simulink model "generic_IVS"  (R2024a)
settings: Solver=FixedStepDiscrete  StartTime=0.0  StopTime=inf  FixedStep=0.001  RelTol=1e-3  EnableMultiTasking=on
libraries: CarMaker4SL x52, slpidlib x2, simulink x1
(part 3 of 3)

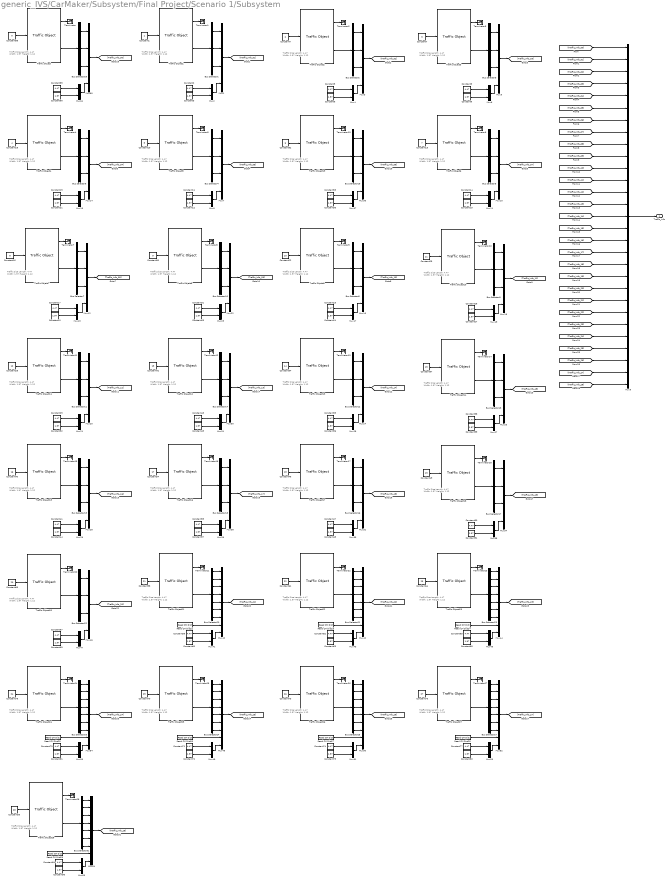
== system generic_IVS/CarMaker/Subsystem/Final Project/Scenario 1/Subsystem ==
  note: Traffic Size
      | Length: 4.47
      | Width: 1.97
      | Height: 1.12
  note: Traffic Size
      | Length: 4.47
      | Width: 1.97
      | Height: 1.12
  note: Traffic Size
      | Length: 4.47
      | Width: 1.97
      | Height: 1.12
  note: Traffic Size
      | Length: 4.47
      | Width: 1.97
      | Height: 1.12
  note: Traffic Size
      | Length: 4.47
      | Width: 1.97
      | Height: 1.12
  note: Traffic Size
      | Length: 4.47
      | Width: 1.97
      | Height: 1.12
  note: Traffic Size
      | Length: 4.47
      | Width: 1.97
      | Height: 1.12
  note: Traffic Size
      | Length: 4.47
      | Width: 1.97
      | Height: 1.12
  note: Traffic Size
      | Length: 4.47
      | Width: 1.97
      | Height: 1.12
  note: Traffic Size
      | Length: 4.47
      | Width: 1.97
      | Height: 1.12
  note: Traffic Size
      | Length: 4.47
      | Width: 1.97
      | Height: 1.12
  note: Traffic Size
      | Length: 4.47
      | Width: 1.97
      | Height: 1.12
  note: Traffic Size
      | Length: 4.47
      | Width: 1.97
      | Height: 1.12
  note: Traffic Size
      | Length: 4.47
      | Width: 1.97
      | Height: 1.12
  note: Traffic Size
      | Length: 4.47
      | Width: 1.97
      | Height: 1.12
  note: Traffic Size
      | Length: 4.47
      | Width: 1.97
      | Height: 1.12
  note: Traffic Size
      | Length: 4.47
      | Width: 1.97
      | Height: 1.12
  note: Traffic Size
      | Length: 4.47
      | Width: 1.97
      | Height: 1.12
  note: Traffic Size
      | Length: 4.47
      | Width: 1.97
      | Height: 1.12
  note: Traffic Size
      | Length: 4.47
      | Width: 1.97
      | Height: 1.12
  note: Traffic Size
      | Length: 4.47
      | Width: 1.97
      | Height: 1.12
  note: Traffic Size
      | Length: 4.47
      | Width: 1.97
      | Height: 1.12
  note: Traffic Size
      | Length: 4.47
      | Width: 1.97
      | Height: 1.12
  note: Traffic Size
      | Length: 4.47
      | Width: 1.97
      | Height: 1.12
  note: Traffic Size
      | Length: 4.47
      | Width: 1.97
      | Height: 1.12
  note: Traffic Size
      | Length: 4.47
      | Width: 1.97
      | Height: 1.12
  note: Traffic Size
      | Length: 4.47
      | Width: 1.97
      | Height: 1.12
  note: Traffic Size
      | Length: 4.47
      | Width: 1.97
      | Height: 1.12
  note: Traffic Size
      | Length: 4.47
      | Width: 1.97
      | Height: 1.12
  Bus Selector{1..19,22,29} (21 alike) : BusSelector  OutputSignals=t_0 x,t_0 y,r_zyx z
  Bus Selector{20..21,23..27,31} (8 alike) : BusSelector  OutputSignals=t_0 x,t_0 y,v_0 x,v_0 y,a_0 x,a_0 y,r_zyx z
  Constant1 : Constant
  Constant10 : Constant  Value=5
  Constant{2,5,8,11,14,17,19,23,26,29,31,35,38,41,43,47,50,53,55,59,62,65,67,71,74,77,79,89,94} (29 alike) : Constant  Value=4.47
  Constant{3,6,9,12,15,20..21,24,27,32..33,36,39,44..45,48,51,56..57,60,63,68..69,72,75,80..81,90,96} (29 alike) : Constant  Value=1.97
  Constant13 : Constant  Value=7
  Constant16 : Constant  Value=8
  Constant18 : Constant  Value=4
  Constant22 : Constant  Value=10
  Constant25 : Constant  Value=11
  Constant28 : Constant  Value=12
  Constant30 : Constant  Value=9
  Constant34 : Constant  Value=14
  Constant37 : Constant  Value=15
  Constant4 : Constant  Value=2
  Constant40 : Constant  Value=16
  Constant42 : Constant  Value=13
  Constant46 : Constant  Value=18
  Constant49 : Constant  Value=19
  Constant52 : Constant  Value=6
  Constant54 : Constant  Value=17
  Constant58 : Constant  Value=21
  Constant61 : Constant  Value=22
  Constant64 : Constant  Value=23
  Constant66 : Constant  Value=20
  Constant7 : Constant  Value=3
  Constant70 : Constant  Value=25
  Constant73 : Constant  Value=26
  Constant76 : Constant  Value=27
  Constant78 : Constant  Value=24
  Constant88 : Constant  Value=0
  Constant93 : Constant  Value=28
  Mux{1,3,5,7,10,12,14,16,18,20,22,24,26,28,30,32,34,36,38,46,60} (21 alike) : Mux
  Mux{2,4,6,8,11,13,15,17,19,21,23,25,27,29,31,33,35,37,39,41,43,45,47,49,51,53,55,61,65} (29 alike) : Mux  Inputs=2
  Mux{40,42,44,48,50,52,54,64} (8 alike) : Mux  Inputs=9
  Mux9 : Mux  Inputs=29
  Read CM Dict22 : CarMaker4SL/Read CM Dict  xname=Traffic.T21.rzv  xsync=off  xstime=Inherited
  Read CM Dict23 : CarMaker4SL/Read CM Dict  xname=Traffic.T22.rzv  xsync=off  xstime=Inherited
  Read CM Dict24 : CarMaker4SL/Read CM Dict  xname=Traffic.T23.rzv  xsync=off  xstime=Inherited
  Read CM Dict25 : CarMaker4SL/Read CM Dict  xname=Traffic.T24.rzv  xsync=off  xstime=Inherited
  Read CM Dict26 : CarMaker4SL/Read CM Dict  xname=Traffic.T25.rzv  xsync=off  xstime=Inherited
  Read CM Dict27 : CarMaker4SL/Read CM Dict  xname=Traffic.T26.rzv  xsync=off  xstime=Inherited
  Read CM Dict28 : CarMaker4SL/Read CM Dict  xname=Traffic.T27.rzv  xsync=off  xstime=Inherited
  Read CM Dict29 : CarMaker4SL/Read CM Dict  xname=Traffic.T28.rzv  xsync=off  xstime=Inherited
  Terminator{,1..28} (29 alike) : Terminator
  Traffic Object : CarMaker4SL/Traffic Object  xname=T00  ximode=Traffic Id  xstime=Inherited
      settings: SourceProductName=CarMaker4SL
  Traffic Object1 : CarMaker4SL/Traffic Object  xname=T01  ximode=Traffic Id  xstime=Inherited
      settings: SourceProductName=CarMaker4SL
  Traffic Object10 : CarMaker4SL/Traffic Object  xname=T11  ximode=Traffic Id  xstime=Inherited
      settings: SourceProductName=CarMaker4SL
  Traffic Object11 : CarMaker4SL/Traffic Object  xname=T12  ximode=Traffic Id  xstime=Inherited
      settings: SourceProductName=CarMaker4SL
  Traffic Object12 : CarMaker4SL/Traffic Object  xname=T13  ximode=Traffic Id  xstime=Inherited
      settings: SourceProductName=CarMaker4SL
  Traffic Object13 : CarMaker4SL/Traffic Object  xname=T14  ximode=Traffic Id  xstime=Inherited
      settings: SourceProductName=CarMaker4SL
  Traffic Object14 : CarMaker4SL/Traffic Object  xname=T15  ximode=Traffic Id  xstime=Inherited
      settings: SourceProductName=CarMaker4SL
  Traffic Object15 : CarMaker4SL/Traffic Object  xname=T16  ximode=Traffic Id  xstime=Inherited
      settings: SourceProductName=CarMaker4SL
  Traffic Object16 : CarMaker4SL/Traffic Object  xname=T17  ximode=Traffic Id  xstime=Inherited
      settings: SourceProductName=CarMaker4SL
  Traffic Object17 : CarMaker4SL/Traffic Object  xname=T18  ximode=Traffic Id  xstime=Inherited
      settings: SourceProductName=CarMaker4SL
  Traffic Object18 : CarMaker4SL/Traffic Object  xname=T19  ximode=Traffic Id  xstime=Inherited
      settings: SourceProductName=CarMaker4SL
  Traffic Object19 : CarMaker4SL/Traffic Object  xname=T06  ximode=Traffic Id  xstime=Inherited
      settings: SourceProductName=CarMaker4SL
  Traffic Object2 : CarMaker4SL/Traffic Object  xname=T02  ximode=Traffic Id  xstime=Inherited
      settings: SourceProductName=CarMaker4SL
  Traffic Object20 : CarMaker4SL/Traffic Object  xname=T20  ximode=Traffic Id  xstime=Inherited
      settings: SourceProductName=CarMaker4SL
  Traffic Object21 : CarMaker4SL/Traffic Object  xname=T21  ximode=Traffic Id  xstime=Inherited
      settings: SourceProductName=CarMaker4SL
  Traffic Object22 : CarMaker4SL/Traffic Object  xname=T22  ximode=Traffic Id  xstime=Inherited
      settings: SourceProductName=CarMaker4SL
  Traffic Object23 : CarMaker4SL/Traffic Object  xname=T23  ximode=Traffic Id  xstime=Inherited
      settings: SourceProductName=CarMaker4SL
  Traffic Object24 : CarMaker4SL/Traffic Object  xname=T24  ximode=Traffic Id  xstime=Inherited
      settings: SourceProductName=CarMaker4SL
  Traffic Object25 : CarMaker4SL/Traffic Object  xname=T25  ximode=Traffic Id  xstime=Inherited
      settings: SourceProductName=CarMaker4SL
  Traffic Object26 : CarMaker4SL/Traffic Object  xname=T26  ximode=Traffic Id  xstime=Inherited
      settings: SourceProductName=CarMaker4SL
  Traffic Object27 : CarMaker4SL/Traffic Object  xname=T27  ximode=Traffic Id  xstime=Inherited
      settings: SourceProductName=CarMaker4SL
  Traffic Object28 : CarMaker4SL/Traffic Object  xname=T28  ximode=Traffic Id  xstime=Inherited
      settings: SourceProductName=CarMaker4SL
  Traffic Object3 : CarMaker4SL/Traffic Object  xname=T03  ximode=Traffic Id  xstime=Inherited
      settings: SourceProductName=CarMaker4SL
  Traffic Object4 : CarMaker4SL/Traffic Object  xname=T04  ximode=Traffic Id  xstime=Inherited
      settings: SourceProductName=CarMaker4SL
  Traffic Object5 : CarMaker4SL/Traffic Object  xname=T05  ximode=Traffic Id  xstime=Inherited
      settings: SourceProductName=CarMaker4SL
  Traffic Object6 : CarMaker4SL/Traffic Object  xname=T07  ximode=Traffic Id  xstime=Inherited
      settings: SourceProductName=CarMaker4SL
  Traffic Object7 : CarMaker4SL/Traffic Object  xname=T08  ximode=Traffic Id  xstime=Inherited
      settings: SourceProductName=CarMaker4SL
  Traffic Object8 : CarMaker4SL/Traffic Object  xname=T09  ximode=Traffic Id  xstime=Inherited
      settings: SourceProductName=CarMaker4SL
  Traffic Object9 : CarMaker4SL/Traffic Object  xname=T10  ximode=Traffic Id  xstime=Inherited
      settings: SourceProductName=CarMaker4SL
  Traffic_Info : Outport
  wires:
  [Traffic_Info_00] -> Mux9/1
  [Traffic_Info_01] -> Mux9/2
  Mux9/1 -> Traffic_Info/1
  [Traffic_Info_02] -> Mux9/3
  [Traffic_Info_06] -> Mux9/7
  [Traffic_Info_05] -> Mux9/6
  [Traffic_Info_04] -> Mux9/5
  [Traffic_Info_03] -> Mux9/4
  [Traffic_Info_09] -> Mux9/10
  [Traffic_Info_10] -> Mux9/11
  [Traffic_Info_11] -> Mux9/12
  [Traffic_Info_08] -> Mux9/9
  [Traffic_Info_12] -> Mux9/13
  [Traffic_Info_13] -> Mux9/14
  [Traffic_Info_07] -> Mux9/8
  [Traffic_Info_16] -> Mux9/17
  [Traffic_Info_17] -> Mux9/18
  [Traffic_Info_18] -> Mux9/19
  [Traffic_Info_15] -> Mux9/16
  [Traffic_Info_19] -> Mux9/20
  [Traffic_Info_20] -> Mux9/21
  [Traffic_Info_14] -> Mux9/15
  [Traffic_Info_23] -> Mux9/24
  [Traffic_Info_24] -> Mux9/25
  [Traffic_Info_25] -> Mux9/26
  [Traffic_Info_22] -> Mux9/23
  [Traffic_Info_26] -> Mux9/27
  [Traffic_Info_27] -> Mux9/28
  [Traffic_Info_21] -> Mux9/22
  [Traffic_Info_28] -> Mux9/29
  Traffic Object/2 -> Bus Selector29/1
  Constant88/1 -> Traffic Object/1
  Traffic Object/1 -> Terminator/1
  Bus Selector29/1 -> Mux60/1  "<t_0 x>"
  Bus Selector29/2 -> Mux60/2  "<t_0 y>"
  Bus Selector29/3 -> Mux60/3  "<r_zyx z>"
  Mux60/1 -> [Traffic_Info_00]
  Constant89/1 -> Mux61/1
  Constant90/1 -> Mux61/2
  Mux61/1 -> Mux60/4
  Bus Selector23/5 -> Mux44/5  "<a_0 x>"
  Traffic Object22/2 -> Bus Selector21/1
  Mux41/1 -> Mux40/9
  Constant63/1 -> Mux43/2
  Bus Selector23/2 -> Mux44/2  "<t_0 y>"
  Bus Selector21/2 -> Mux42/2  "<t_0 y>"
  Bus Selector21/5 -> Mux42/5  "<a_0 x>"
  Traffic Object22/1 -> Terminator22/1
  Bus Selector23/6 -> Mux44/6  "<a_0 y>"
  Bus Selector23/7 -> Mux44/7  "<r_zyx z>"
  Traffic Object23/1 -> Terminator23/1
  Traffic Object23/2 -> Bus Selector23/1
  Constant68/1 -> Mux45/2
  Mux45/1 -> Mux44/9
  Constant61/1 -> Traffic Object22/1
  Read CM Dict24/1 -> Mux44/8
  Mux42/1 -> [Traffic_Info_22]
  Mux40/1 -> [Traffic_Info_21]
  Mux44/1 -> [Traffic_Info_23]
  Bus Selector23/4 -> Mux44/4  "<v_0 y>"
  Bus Selector21/6 -> Mux42/6  "<a_0 y>"
  Bus Selector20/6 -> Mux40/6  "<a_0 y>"
  Bus Selector21/3 -> Mux42/3  "<v_0 x>"
  Bus Selector21/4 -> Mux42/4  "<v_0 y>"
  Bus Selector21/1 -> Mux42/1  "<t_0 x>"
  Constant58/1 -> Traffic Object21/1
  Bus Selector21/7 -> Mux42/7  "<r_zyx z>"
  Constant65/1 -> Mux45/1
  Bus Selector20/1 -> Mux40/1  "<t_0 x>"
  Bus Selector23/1 -> Mux44/1  "<t_0 x>"
  Bus Selector20/3 -> Mux40/3  "<v_0 x>"
  Constant60/1 -> Mux41/2
  Traffic Object21/2 -> Bus Selector20/1
  Read CM Dict22/1 -> Mux40/8
  Bus Selector20/5 -> Mux40/5  "<a_0 x>"
  Traffic Object21/1 -> Terminator21/1
  Bus Selector20/2 -> Mux40/2  "<t_0 y>"
  Bus Selector23/3 -> Mux44/3  "<v_0 x>"
  Constant64/1 -> Traffic Object23/1
  Bus Selector20/7 -> Mux40/7  "<r_zyx z>"
  Read CM Dict23/1 -> Mux42/8
  Constant62/1 -> Mux43/1
  Bus Selector20/4 -> Mux40/4  "<v_0 y>"
  Constant59/1 -> Mux41/1
  Mux43/1 -> Mux42/9
  Bus Selector26/3 -> Mux54/3  "<v_0 x>"
  Bus Selector27/5 -> Mux52/5  "<a_0 x>"
  Bus Selector26/5 -> Mux54/5  "<a_0 x>"
  Traffic Object26/2 -> Bus Selector25/1
  Bus Selector26/6 -> Mux54/6  "<a_0 y>"
  Mux49/1 -> Mux48/9
  Constant75/1 -> Mux51/2
  Bus Selector27/2 -> Mux52/2  "<t_0 y>"
  Bus Selector25/2 -> Mux50/2  "<t_0 y>"
  Bus Selector25/5 -> Mux50/5  "<a_0 x>"
  Traffic Object26/1 -> Terminator26/1
  Bus Selector27/6 -> Mux52/6  "<a_0 y>"
  Bus Selector26/7 -> Mux54/7  "<r_zyx z>"
  Bus Selector27/7 -> Mux52/7  "<r_zyx z>"
  Bus Selector26/1 -> Mux54/1  "<t_0 x>"
  Traffic Object27/1 -> Terminator27/1
  Traffic Object27/2 -> Bus Selector27/1
  Constant80/1 -> Mux53/2
  Mux53/1 -> Mux52/9
  Constant73/1 -> Traffic Object26/1
  Read CM Dict28/1 -> Mux52/8
  Mux50/1 -> [Traffic_Info_26]
  Mux48/1 -> [Traffic_Info_25]
  Mux52/1 -> [Traffic_Info_27]
  Bus Selector27/4 -> Mux52/4  "<v_0 y>"
  Constant78/1 -> Traffic Object24/1
  Traffic Object24/1 -> Terminator24/1
  Bus Selector25/6 -> Mux50/6  "<a_0 y>"
  Bus Selector24/6 -> Mux48/6  "<a_0 y>"
  Bus Selector25/3 -> Mux50/3  "<v_0 x>"
  Read CM Dict25/1 -> Mux54/8
  Bus Selector25/4 -> Mux50/4  "<v_0 y>"
  Bus Selector26/4 -> Mux54/4  "<v_0 y>"
  Bus Selector25/1 -> Mux50/1  "<t_0 x>"
  Constant70/1 -> Traffic Object25/1
  Bus Selector25/7 -> Mux50/7  "<r_zyx z>"
  Constant77/1 -> Mux53/1
  Bus Selector26/2 -> Mux54/2  "<t_0 y>"
  Bus Selector24/1 -> Mux48/1  "<t_0 x>"
  Bus Selector27/1 -> Mux52/1  "<t_0 x>"
  Bus Selector24/3 -> Mux48/3  "<v_0 x>"
  Mux54/1 -> [Traffic_Info_24]
  Constant72/1 -> Mux49/2
  Traffic Object25/2 -> Bus Selector24/1
  Read CM Dict26/1 -> Mux48/8
  Bus Selector24/5 -> Mux48/5  "<a_0 x>"
  Traffic Object25/1 -> Terminator25/1
  Constant81/1 -> Mux55/2
  Bus Selector24/2 -> Mux48/2  "<t_0 y>"
  Bus Selector27/3 -> Mux52/3  "<v_0 x>"
  Constant76/1 -> Traffic Object27/1
  Bus Selector24/7 -> Mux48/7  "<r_zyx z>"
  Traffic Object24/2 -> Bus Selector26/1
  Read CM Dict27/1 -> Mux50/8
  Mux55/1 -> Mux54/9
  Constant74/1 -> Mux51/1
  Bus Selector24/4 -> Mux48/4  "<v_0 y>"
  Constant71/1 -> Mux49/1
  Constant79/1 -> Mux55/1
  Mux51/1 -> Mux50/9
  Bus Selector31/3 -> Mux64/3  "<v_0 x>"
  Bus Selector31/5 -> Mux64/5  "<a_0 x>"
  Bus Selector31/6 -> Mux64/6  "<a_0 y>"
  Bus Selector31/7 -> Mux64/7  "<r_zyx z>"
  Bus Selector31/1 -> Mux64/1  "<t_0 x>"
  Constant93/1 -> Traffic Object28/1
  Traffic Object28/1 -> Terminator28/1
  Read CM Dict29/1 -> Mux64/8
  Bus Selector31/4 -> Mux64/4  "<v_0 y>"
  Bus Selector31/2 -> Mux64/2  "<t_0 y>"
  Mux64/1 -> [Traffic_Info_28]
  Constant96/1 -> Mux65/2
  Traffic Object28/2 -> Bus Selector31/1
  Mux65/1 -> Mux64/9
  Constant94/1 -> Mux65/1
  Bus Selector1/3 -> Mux1/3  "<r_zyx z>"
  Mux1/1 -> [Traffic_Info_01]
  Bus Selector1/1 -> Mux1/1  "<t_0 x>"
  Traffic Object1/1 -> Terminator1/1
  Constant2/1 -> Mux2/1
  Constant3/1 -> Mux2/2
  Bus Selector1/2 -> Mux1/2  "<t_0 y>"
  Mux2/1 -> Mux1/4
  Constant1/1 -> Traffic Object1/1
  Traffic Object1/2 -> Bus Selector1/1
  Bus Selector2/3 -> Mux3/3  "<r_zyx z>"
  Mux3/1 -> [Traffic_Info_02]
  Bus Selector2/1 -> Mux3/1  "<t_0 x>"
  Traffic Object2/1 -> Terminator2/1
  Constant5/1 -> Mux4/1
  Constant6/1 -> Mux4/2
  Bus Selector2/2 -> Mux3/2  "<t_0 y>"
  Mux4/1 -> Mux3/4
  Constant4/1 -> Traffic Object2/1
  Traffic Object2/2 -> Bus Selector2/1
  Bus Selector3/3 -> Mux5/3  "<r_zyx z>"
  Mux5/1 -> [Traffic_Info_03]
  Bus Selector3/1 -> Mux5/1  "<t_0 x>"
  Traffic Object3/1 -> Terminator3/1
  Constant8/1 -> Mux6/1
  Constant9/1 -> Mux6/2
  Bus Selector3/2 -> Mux5/2  "<t_0 y>"
  Mux6/1 -> Mux5/4
  Constant7/1 -> Traffic Object3/1
  Traffic Object3/2 -> Bus Selector3/1
  Bus Selector6/3 -> Mux14/3  "<r_zyx z>"
  Mux14/1 -> [Traffic_Info_04]
  Bus Selector6/1 -> Mux14/1  "<t_0 x>"
  Mux8/1 -> Mux7/4
  Constant12/1 -> Mux8/2
  Mux7/1 -> [Traffic_Info_05]
  Traffic Object4/1 -> Terminator4/1
  Bus Selector4/2 -> Mux7/2  "<t_0 y>"
  Constant18/1 -> Traffic Object4/1
  Constant21/1 -> Mux15/2
  Constant10/1 -> Traffic Object5/1
  Bus Selector6/2 -> Mux14/2  "<t_0 y>"
  Mux15/1 -> Mux14/4
  Traffic Object4/2 -> Bus Selector6/1
  Constant16/1 -> Traffic Object7/1
  Traffic Object7/2 -> Bus Selector7/1
  Constant17/1 -> Mux13/1
  Constant19/1 -> Mux15/1
  Constant11/1 -> Mux8/1
  Traffic Object7/1 -> Terminator7/1
  Constant20/1 -> Mux13/2
  Bus Selector4/1 -> Mux7/1  "<t_0 x>"
  Mux13/1 -> Mux12/4
  Bus Selector7/1 -> Mux12/1  "<t_0 x>"
  Bus Selector4/3 -> Mux7/3  "<r_zyx z>"
  Bus Selector7/3 -> Mux12/3  "<r_zyx z>"
  Mux12/1 -> [Traffic_Info_08]
  Constant15/1 -> Mux11/2
  Mux11/1 -> Mux10/4
  Constant13/1 -> Traffic Object6/1
  Traffic Object5/1 -> Terminator5/1
  Constant14/1 -> Mux11/1
  Traffic Object6/1 -> Terminator6/1
  Traffic Object5/2 -> Bus Selector4/1
  Bus Selector5/1 -> Mux10/1  "<t_0 x>"
  Bus Selector7/2 -> Mux12/2  "<t_0 y>"
  Traffic Object6/2 -> Bus Selector5/1
  Bus Selector5/3 -> Mux10/3  "<r_zyx z>"
  Mux10/1 -> [Traffic_Info_07]
  Bus Selector5/2 -> Mux10/2  "<t_0 y>"
  Bus Selector10/3 -> Mux22/3  "<r_zyx z>"
  Mux22/1 -> [Traffic_Info_09]
  Bus Selector10/1 -> Mux22/1  "<t_0 x>"
  Mux17/1 -> Mux16/4
  Constant24/1 -> Mux17/2
  Mux16/1 -> [Traffic_Info_10]
  Traffic Object8/1 -> Terminator8/1
  Bus Selector8/2 -> Mux16/2  "<t_0 y>"
  Constant30/1 -> Traffic Object8/1
  Constant33/1 -> Mux23/2
  Constant22/1 -> Traffic Object9/1
  Bus Selector10/2 -> Mux22/2  "<t_0 y>"
  Mux23/1 -> Mux22/4
  Traffic Object8/2 -> Bus Selector10/1
  Constant28/1 -> Traffic Object11/1
  Traffic Object11/2 -> Bus Selector11/1
  Constant29/1 -> Mux21/1
  Constant31/1 -> Mux23/1
  Constant23/1 -> Mux17/1
  Traffic Object11/1 -> Terminator11/1
  Constant32/1 -> Mux21/2
  Bus Selector8/1 -> Mux16/1  "<t_0 x>"
  Mux21/1 -> Mux20/4
  Bus Selector11/1 -> Mux20/1  "<t_0 x>"
  Bus Selector8/3 -> Mux16/3  "<r_zyx z>"
  Bus Selector11/3 -> Mux20/3  "<r_zyx z>"
  Mux20/1 -> [Traffic_Info_12]
  Constant27/1 -> Mux19/2
  Mux19/1 -> Mux18/4
  Constant25/1 -> Traffic Object10/1
  Traffic Object9/1 -> Terminator9/1
  Constant26/1 -> Mux19/1
  Traffic Object10/1 -> Terminator10/1
  Traffic Object9/2 -> Bus Selector8/1
  Bus Selector9/1 -> Mux18/1  "<t_0 x>"
  Bus Selector11/2 -> Mux20/2  "<t_0 y>"
  Traffic Object10/2 -> Bus Selector9/1
  Bus Selector9/3 -> Mux18/3  "<r_zyx z>"
  Mux18/1 -> [Traffic_Info_11]
  Bus Selector9/2 -> Mux18/2  "<t_0 y>"
  Bus Selector14/3 -> Mux30/3  "<r_zyx z>"
  Mux30/1 -> [Traffic_Info_13]
  Bus Selector14/1 -> Mux30/1  "<t_0 x>"
  Mux25/1 -> Mux24/4
  Constant36/1 -> Mux25/2
  Mux24/1 -> [Traffic_Info_14]
  Traffic Object12/1 -> Terminator12/1
  Bus Selector12/2 -> Mux24/2  "<t_0 y>"
  Constant42/1 -> Traffic Object12/1
  Constant45/1 -> Mux31/2
  Constant34/1 -> Traffic Object13/1
  Bus Selector14/2 -> Mux30/2  "<t_0 y>"
  Mux31/1 -> Mux30/4
  Traffic Object12/2 -> Bus Selector14/1
  Constant40/1 -> Traffic Object15/1
  Traffic Object15/2 -> Bus Selector15/1
  Constant41/1 -> Mux29/1
  Constant43/1 -> Mux31/1
  Constant35/1 -> Mux25/1
  Traffic Object15/1 -> Terminator15/1
  Constant44/1 -> Mux29/2
  Bus Selector12/1 -> Mux24/1  "<t_0 x>"
  Mux29/1 -> Mux28/4
  Bus Selector15/1 -> Mux28/1  "<t_0 x>"
  Bus Selector12/3 -> Mux24/3  "<r_zyx z>"
  Bus Selector15/3 -> Mux28/3  "<r_zyx z>"
  Mux28/1 -> [Traffic_Info_16]
  Constant39/1 -> Mux27/2
  Mux27/1 -> Mux26/4
  Constant37/1 -> Traffic Object14/1
  Traffic Object13/1 -> Terminator13/1
  Constant38/1 -> Mux27/1
  Traffic Object14/1 -> Terminator14/1
  Traffic Object13/2 -> Bus Selector12/1
  Bus Selector13/1 -> Mux26/1  "<t_0 x>"
  Bus Selector15/2 -> Mux28/2  "<t_0 y>"
  Traffic Object14/2 -> Bus Selector13/1
  Bus Selector13/3 -> Mux26/3  "<r_zyx z>"
  Mux26/1 -> [Traffic_Info_15]
  Bus Selector13/2 -> Mux26/2  "<t_0 y>"
  Bus Selector17/1 -> Mux34/1  "<t_0 x>"
  Traffic Object18/1 -> Terminator18/1
  Constant49/1 -> Traffic Object18/1
  Traffic Object17/2 -> Bus Selector16/1
  Traffic Object17/1 -> Terminator17/1
  Mux34/1 -> [Traffic_Info_19]
  Bus Selector17/3 -> Mux34/3  "<r_zyx z>"
  Constant50/1 -> Mux35/1
  Constant51/1 -> Mux35/2
  Traffic Object18/2 -> Bus Selector17/1
  Constant55/1 -> Mux39/1
  Bus Selector17/2 -> Mux34/2  "<t_0 y>"
  Constant47/1 -> Mux33/1
  Bus Selector16/1 -> Mux32/1  "<t_0 x>"
  Bus Selector16/3 -> Mux32/3  "<r_zyx z>"
  Traffic Object16/2 -> Bus Selector18/1
  Mux39/1 -> Mux38/4
  Constant46/1 -> Traffic Object17/1
  Mux35/1 -> Mux34/4
  Mux32/1 -> [Traffic_Info_18]
  Constant54/1 -> Traffic Object16/1
  Traffic Object16/1 -> Terminator16/1
  Constant48/1 -> Mux33/2
  Mux33/1 -> Mux32/4
  Constant57/1 -> Mux39/2
  Bus Selector18/1 -> Mux38/1  "<t_0 x>"
  Bus Selector18/3 -> Mux38/3  "<r_zyx z>"
  Bus Selector16/2 -> Mux32/2  "<t_0 y>"
  Mux38/1 -> [Traffic_Info_17]
  Bus Selector18/2 -> Mux38/2  "<t_0 y>"
  Bus Selector19/1 -> Mux36/1  "<t_0 x>"
  Traffic Object19/1 -> Terminator19/1
  Constant53/1 -> Mux37/1
  Bus Selector19/2 -> Mux36/2  "<t_0 y>"
  Mux36/1 -> [Traffic_Info_06]
  Bus Selector19/3 -> Mux36/3  "<r_zyx z>"
  Traffic Object19/2 -> Bus Selector19/1
  Mux37/1 -> Mux36/4
  Constant52/1 -> Traffic Object19/1
  Constant56/1 -> Mux37/2
  Constant69/1 -> Mux47/2
  Traffic Object20/2 -> Bus Selector22/1
  Bus Selector22/2 -> Mux46/2  "<t_0 y>"
  Bus Selector22/3 -> Mux46/3  "<r_zyx z>"
  Mux46/1 -> [Traffic_Info_20]
  Constant67/1 -> Mux47/1
  Mux47/1 -> Mux46/4
  Bus Selector22/1 -> Mux46/1  "<t_0 x>"
  Constant66/1 -> Traffic Object20/1
  Traffic Object20/1 -> Terminator20/1

== system generic_IVS/CarMaker/IPG Vehicle/CarAndTrailer/Forces/Suspension Forces/Suspension External Forces Update ==
  Bus Creator21 : BusCreator  Inputs=6
  Bus Creator22 : BusCreator  Inputs=4
  Bus Creator23 : BusCreator  Inputs=4
  From : From  TagVisibility=global
  Ground{32..39} (8 alike) : Ground
  Out1 : Outport
  wires:
  [D] -> Bus Creator21/4
  Ground36/1 -> Bus Creator22/1
  From/1 -> Bus Creator21/1
  [B] -> Bus Creator21/2
  Ground34/1 -> Bus Creator23/3
  Ground32/1 -> Bus Creator23/1
  [C] -> Bus Creator21/3
  Bus Creator23/1 -> Bus Creator21/5
  Ground33/1 -> Bus Creator23/2
  Bus Creator22/1 -> Bus Creator21/6
  Bus Creator21/1 -> Out1/1
  Ground35/1 -> Bus Creator23/4
  Ground39/1 -> Bus Creator22/4
  Ground38/1 -> Bus Creator22/3
  Ground37/1 -> Bus Creator22/2

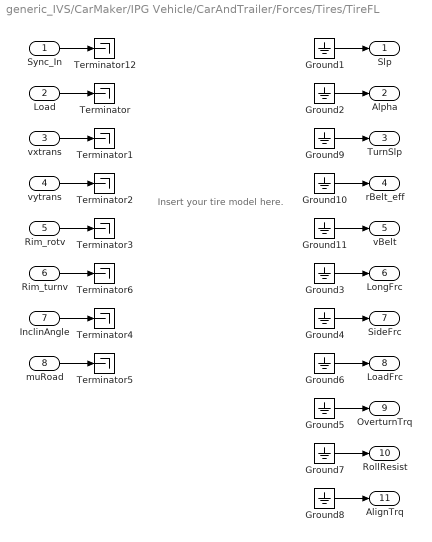
== system generic_IVS/CarMaker/IPG Vehicle/CarAndTrailer/Forces/Tires/TireFL ==
  note: Insert your tire model here.
  Sync_In : Inport
  Load : Inport  Port=2
  vxtrans : Inport  Port=3
  vytrans : Inport  Port=4
  Rim_rotv : Inport  Port=5
  Rim_turnv : Inport  Port=6
  InclinAngle : Inport  Port=7
  muRoad : Inport  Port=8
  Ground{1..11} (11 alike) : Ground
  Terminator{,1..6,12} (8 alike) : Terminator
  Slp : Outport  VectorParamsAs1DForOutWhenUnconnected=off
  Alpha : Outport  Port=2  VectorParamsAs1DForOutWhenUnconnected=off
  TurnSlp : Outport  Port=3  VectorParamsAs1DForOutWhenUnconnected=off
  rBelt_eff : Outport  Port=4  VectorParamsAs1DForOutWhenUnconnected=off
  vBelt : Outport  Port=5  VectorParamsAs1DForOutWhenUnconnected=off
  LongFrc : Outport  Port=6  VectorParamsAs1DForOutWhenUnconnected=off
  SideFrc : Outport  Port=7  VectorParamsAs1DForOutWhenUnconnected=off
  LoadFrc : Outport  Port=8  VectorParamsAs1DForOutWhenUnconnected=off
  OverturnTrq : Outport  Port=9  VectorParamsAs1DForOutWhenUnconnected=off
  RollResist : Outport  Port=10  VectorParamsAs1DForOutWhenUnconnected=off
  AlignTrq : Outport  Port=11  VectorParamsAs1DForOutWhenUnconnected=off
  wires:
  Ground11/1 -> vBelt/1
  Ground10/1 -> rBelt_eff/1
  Ground9/1 -> TurnSlp/1
  Rim_turnv/1 -> Terminator6/1
  Sync_In/1 -> Terminator12/1
  Ground2/1 -> Alpha/1
  Ground3/1 -> LongFrc/1
  Ground4/1 -> SideFrc/1
  Ground5/1 -> OverturnTrq/1
  vxtrans/1 -> Terminator1/1
  vytrans/1 -> Terminator2/1
  Rim_rotv/1 -> Terminator3/1
  InclinAngle/1 -> Terminator4/1
  muRoad/1 -> Terminator5/1
  Load/1 -> Terminator/1
  Ground1/1 -> Slp/1
  Ground6/1 -> LoadFrc/1
  Ground7/1 -> RollResist/1
  Ground8/1 -> AlignTrq/1

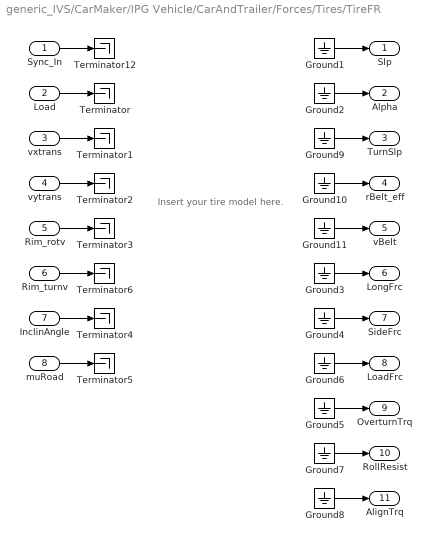
== system generic_IVS/CarMaker/IPG Vehicle/CarAndTrailer/Forces/Tires/TireFR ==
  note: Insert your tire model here.
  Sync_In : Inport
  Load : Inport  Port=2
  vxtrans : Inport  Port=3
  vytrans : Inport  Port=4
  Rim_rotv : Inport  Port=5
  Rim_turnv : Inport  Port=6
  InclinAngle : Inport  Port=7
  muRoad : Inport  Port=8
  Ground{1..11} (11 alike) : Ground
  Terminator{,1..6,12} (8 alike) : Terminator
  Slp : Outport  VectorParamsAs1DForOutWhenUnconnected=off
  Alpha : Outport  Port=2  VectorParamsAs1DForOutWhenUnconnected=off
  TurnSlp : Outport  Port=3  VectorParamsAs1DForOutWhenUnconnected=off
  rBelt_eff : Outport  Port=4  VectorParamsAs1DForOutWhenUnconnected=off
  vBelt : Outport  Port=5  VectorParamsAs1DForOutWhenUnconnected=off
  LongFrc : Outport  Port=6  VectorParamsAs1DForOutWhenUnconnected=off
  SideFrc : Outport  Port=7  VectorParamsAs1DForOutWhenUnconnected=off
  LoadFrc : Outport  Port=8  VectorParamsAs1DForOutWhenUnconnected=off
  OverturnTrq : Outport  Port=9  VectorParamsAs1DForOutWhenUnconnected=off
  RollResist : Outport  Port=10  VectorParamsAs1DForOutWhenUnconnected=off
  AlignTrq : Outport  Port=11  VectorParamsAs1DForOutWhenUnconnected=off
  wires:
  Ground11/1 -> vBelt/1
  Ground10/1 -> rBelt_eff/1
  Ground9/1 -> TurnSlp/1
  Rim_turnv/1 -> Terminator6/1
  Sync_In/1 -> Terminator12/1
  Ground2/1 -> Alpha/1
  Ground3/1 -> LongFrc/1
  Ground4/1 -> SideFrc/1
  Ground5/1 -> OverturnTrq/1
  vxtrans/1 -> Terminator1/1
  vytrans/1 -> Terminator2/1
  Rim_rotv/1 -> Terminator3/1
  InclinAngle/1 -> Terminator4/1
  muRoad/1 -> Terminator5/1
  Load/1 -> Terminator/1
  Ground1/1 -> Slp/1
  Ground6/1 -> LoadFrc/1
  Ground7/1 -> RollResist/1
  Ground8/1 -> AlignTrq/1

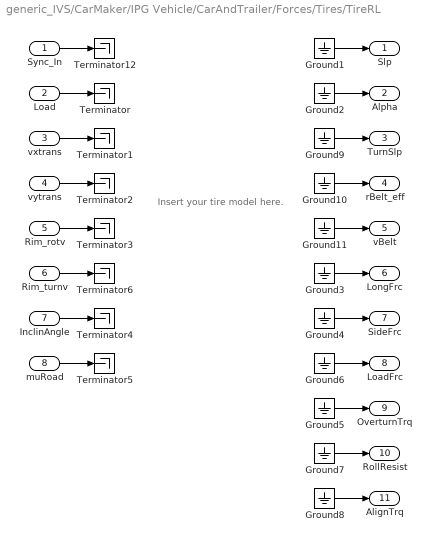
== system generic_IVS/CarMaker/IPG Vehicle/CarAndTrailer/Forces/Tires/TireRL ==
  note: Insert your tire model here.
  Sync_In : Inport
  Load : Inport  Port=2
  vxtrans : Inport  Port=3
  vytrans : Inport  Port=4
  Rim_rotv : Inport  Port=5
  Rim_turnv : Inport  Port=6
  InclinAngle : Inport  Port=7
  muRoad : Inport  Port=8
  Ground{1..11} (11 alike) : Ground
  Terminator{,1..6,12} (8 alike) : Terminator
  Slp : Outport  VectorParamsAs1DForOutWhenUnconnected=off
  Alpha : Outport  Port=2  VectorParamsAs1DForOutWhenUnconnected=off
  TurnSlp : Outport  Port=3  VectorParamsAs1DForOutWhenUnconnected=off
  rBelt_eff : Outport  Port=4  VectorParamsAs1DForOutWhenUnconnected=off
  vBelt : Outport  Port=5  VectorParamsAs1DForOutWhenUnconnected=off
  LongFrc : Outport  Port=6  VectorParamsAs1DForOutWhenUnconnected=off
  SideFrc : Outport  Port=7  VectorParamsAs1DForOutWhenUnconnected=off
  LoadFrc : Outport  Port=8  VectorParamsAs1DForOutWhenUnconnected=off
  OverturnTrq : Outport  Port=9  VectorParamsAs1DForOutWhenUnconnected=off
  RollResist : Outport  Port=10  VectorParamsAs1DForOutWhenUnconnected=off
  AlignTrq : Outport  Port=11  VectorParamsAs1DForOutWhenUnconnected=off
  wires:
  Ground11/1 -> vBelt/1
  Ground10/1 -> rBelt_eff/1
  Ground9/1 -> TurnSlp/1
  Rim_turnv/1 -> Terminator6/1
  Sync_In/1 -> Terminator12/1
  Ground2/1 -> Alpha/1
  Ground3/1 -> LongFrc/1
  Ground4/1 -> SideFrc/1
  Ground5/1 -> OverturnTrq/1
  vxtrans/1 -> Terminator1/1
  vytrans/1 -> Terminator2/1
  Rim_rotv/1 -> Terminator3/1
  InclinAngle/1 -> Terminator4/1
  muRoad/1 -> Terminator5/1
  Load/1 -> Terminator/1
  Ground1/1 -> Slp/1
  Ground6/1 -> LoadFrc/1
  Ground7/1 -> RollResist/1
  Ground8/1 -> AlignTrq/1

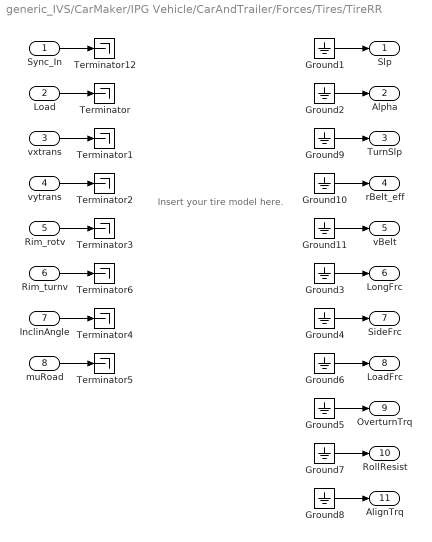
== system generic_IVS/CarMaker/IPG Vehicle/CarAndTrailer/Forces/Tires/TireRR ==
  note: Insert your tire model here.
  Sync_In : Inport
  Load : Inport  Port=2
  vxtrans : Inport  Port=3
  vytrans : Inport  Port=4
  Rim_rotv : Inport  Port=5
  Rim_turnv : Inport  Port=6
  InclinAngle : Inport  Port=7
  muRoad : Inport  Port=8
  Ground{1..11} (11 alike) : Ground
  Terminator{,1..6,12} (8 alike) : Terminator
  Slp : Outport  VectorParamsAs1DForOutWhenUnconnected=off
  Alpha : Outport  Port=2  VectorParamsAs1DForOutWhenUnconnected=off
  TurnSlp : Outport  Port=3  VectorParamsAs1DForOutWhenUnconnected=off
  rBelt_eff : Outport  Port=4  VectorParamsAs1DForOutWhenUnconnected=off
  vBelt : Outport  Port=5  VectorParamsAs1DForOutWhenUnconnected=off
  LongFrc : Outport  Port=6  VectorParamsAs1DForOutWhenUnconnected=off
  SideFrc : Outport  Port=7  VectorParamsAs1DForOutWhenUnconnected=off
  LoadFrc : Outport  Port=8  VectorParamsAs1DForOutWhenUnconnected=off
  OverturnTrq : Outport  Port=9  VectorParamsAs1DForOutWhenUnconnected=off
  RollResist : Outport  Port=10  VectorParamsAs1DForOutWhenUnconnected=off
  AlignTrq : Outport  Port=11  VectorParamsAs1DForOutWhenUnconnected=off
  wires:
  Ground11/1 -> vBelt/1
  Ground10/1 -> rBelt_eff/1
  Ground9/1 -> TurnSlp/1
  Rim_turnv/1 -> Terminator6/1
  Sync_In/1 -> Terminator12/1
  Ground2/1 -> Alpha/1
  Ground3/1 -> LongFrc/1
  Ground4/1 -> SideFrc/1
  Ground5/1 -> OverturnTrq/1
  vxtrans/1 -> Terminator1/1
  vytrans/1 -> Terminator2/1
  Rim_rotv/1 -> Terminator3/1
  InclinAngle/1 -> Terminator4/1
  muRoad/1 -> Terminator5/1
  Load/1 -> Terminator/1
  Ground1/1 -> Slp/1
  Ground6/1 -> LoadFrc/1
  Ground7/1 -> RollResist/1
  Ground8/1 -> AlignTrq/1

== matlab function generic_IVS/CarMaker/Subsystem/Final Project/Scenario 1/MATLAB Function ==
  settings: updateMethod=DISCRETE  sampleTime=1
  data: waypoints_x input; waypoints_y input; X_ego input; Y_ego input; head input; steering_angle output; goal_pose input; speed output
function [steering_angle, speed] = ...
    global_to_local_waypoints(waypoints_x, waypoints_y, ...
                              X_ego, Y_ego, head, goal_pose)
%#codegen
% 글로벌 웨이포인트 → 로컬 좌표 변환 + 조향각 계산 (Pure Pursuit)
% 후방 포인트는 무시하며, 초기에는 아무 유효 포인트 없을 수 있음

    %% 파라미터
    L = 4.0;               % 휠베이스
    epsilon = 1e-3;        % 안정화용
    lookahead_dist = 1.0;  % 추적 기준 거리
    stop_threshold = 2.8;  % 완전 정지 거리
    heading_align_threshold = 15.0;  % 헤딩 조정 시작 거리

    %% 초기값 설정 (모든 실행 경로 보장)
    local_point = [0 0];
    dist = 0;
    idx_closest = 1;
    steering_angle = 0;
    goal_dist = norm([X_ego - goal_pose(1), Y_ego - goal_pose(2)]);
    
    %% 정지 조건
    if goal_dist < stop_threshold
        speed = 0;
        steering_angle = 0;
        return;
    end

    %% 헤딩 정렬 조건 적용
    if goal_dist < heading_align_threshold
        heading_error = wrapToPi(pi/2 - head);  % 90도 방향으로 정렬
        steering_angle = atan2(2 * L * sin(heading_error), goal_dist + epsilon);
        speed = 0;
        % 이 부분에서 
        return;
    end

    %% 1) NaN 제거
    valid_idx = ~isnan(waypoints_x) & ~isnan(waypoints_y);
    x_wp = waypoints_x(valid_idx);
    y_wp = waypoints_y(valid_idx);
    N = numel(x_wp);

    if N == 0
        speed = 0;
        return;
    end

    %% 2) 차량 기준 상대 위치 계산
    dx_all = x_wp(:)' - X_ego;
    dy_all = y_wp(:)' - Y_ego;

    %% 3) 차량 전방 필터
    forward_vec = [cos(head); sin(head)];
    rel_pos = [dx_all; dy_all];
    dot_products = forward_vec' * rel_pos;
    is_in_front = dot_products > 0;

    %% 4) 전방 포인트가 없다면: 정지 상태 유지
    if ~any(is_in_front)
        speed = 0;
        return;
    end

    %% 5) 가장 가까운 전방 인덱스 찾기
    d2_all = dx_all.^2 + dy_all.^2;
    d2_all(~is_in_front) = Inf;
    [~, idx_closest] = min(d2_all);

    %% 6) 전체 로컬 좌표 변환
    c = cos(-head); s = sin(-head);
    R = [c, -s; s, c];
    rel_global = [x_wp - X_ego, y_wp - Y_ego]';
    local_wp = R * rel_global;       % 2×N
    Local_Waypoints = local_wp';     % Nx2
    local_point = Local_Waypoints(idx_closest, :);
    dist = sqrt(d2_all(idx_closest));

    %% 7) 추적 포인트 찾기 (lookahead 거리 기준)
    target_idx = idx_closest;
    for i = idx_closest+1:N
        d = norm(Local_Waypoints(i,:) - Local_Waypoints(idx_closest,:));
        if d > lookahead_dist
            target_idx = i;
            break;
        end
    end

    %% 8) 조향각 계산 (Pure Pursuit)
    x_t = Local_Waypoints(target_idx, 1);
    y_t = Local_Waypoints(target_idx, 2);
    L_d = sqrt(x_t^2 + y_t^2 + epsilon);
    alpha = atan2(y_t, x_t);
    steering_angle = atan2(2 * L * sin(alpha), L_d);

    %% 9) 속도 설정
    speed = 10;
end

%% ===== 각도 wrap =====
function angle = wrapToPi(theta)
    angle = mod(theta + pi, 2*pi) - pi;
end

== matlab function generic_IVS/CarMaker/Subsystem/Final Project/Scenario 1/MATLAB Function3 ==
  settings: updateMethod=DISCRETE  sampleTime=1
  data: map_boundary input; mapMatrix output size=[1000, 1000]; traffic_info input
%% ======== generate_map_ ======== Ver 2025-05-17 10:40
function mapMatrix  = generate_map_(map_boundary, traffic_info)
    %변수설정
    resolution = 0.05;
    traffic_info_mat = reshape(traffic_info(1:5*21), 5, []).';
    x_values = map_boundary(1:2:end);
    y_values = map_boundary(2:2:end);
    N = size(traffic_info_mat,1);
    x_min = min(x_values);  x_max = max(x_values);
    y_min = min(y_values);  y_max = max(y_values);
    x_size = ceil((x_max-x_min)/resolution);
    y_size = ceil((y_max-y_min)/resolution);
    
    
    mapMatrix = zeros(y_size, x_size); %출력코드
    
    for i = 1:N
        x_c = traffic_info_mat(i, 1);
        y_c = traffic_info_mat(i, 2);
        yaw = traffic_info_mat(i, 3);
        length = traffic_info_mat(i, 4);
        width = traffic_info_mat(i, 5);
        
        dx = length/2;  dy = width/2;
        local = [-dx,-dy; dx,-dy; dx,dy; -dx,dy];
        R = [cos(yaw), -sin(yaw); sin(yaw), cos(yaw)];
        rotated = (R*local')';
        forward_vec = [cos(yaw), sin(yaw)];
        side_vec    = [-sin(yaw), cos(yaw)];
        center = [x_c, y_c] + (length/2)*forward_vec - (width/2)*side_vec;
        corners = rotated + center;
        x_idx = (corners(:,1)-x_min)/resolution + 1;
        y_idx = (y_max-corners(:,2))/resolution + 1;
        mask = poly2mask(x_idx, y_idx, y_size, x_size);
        mapMatrix(mask) = 1;
    end
end

== matlab function generic_IVS/CarMaker/Subsystem/Final Project/Scenario 1/MATLAB Function4 ==
  settings: updateMethod=DISCRETE  sampleTime=1
  data: map input; x_path output; startPose input; goalPose input; y_path output; mapboundary input
function [x_path, y_path] = rrt_star_planner(map, startPose, goalPose, mapboundary)
    %% ===== Persistent 저장 =====
    persistent path_initialized x_path_cached y_path_cached nPath_cached
    maxPathLength = 1000;
    resolution = 1;

    if isempty(path_initialized)
        path_initialized = false;
        x_path_cached = zeros(maxPathLength, 1);
        y_path_cached = zeros(maxPathLength, 1);
        nPath_cached = 1;
    end

    if path_initialized
        x_path = x_path_cached(1:nPath_cached);
        y_path = y_path_cached(1:nPath_cached);
        return;
    end

    %% 설정
    visualize      = false;
    maxIter        = 5000;
    stepSize       = 2;
    goalSampleRate = 0.1;
    successDistTh  = 5;
    collisionRes   = 0.5;
    searchRadius   = 5;
    safetyDist     = 0;

    %% 바운더리 기반 인덱스 변환용 파라미터
    x_values = mapboundary(1:2:end);
    y_values = mapboundary(2:2:end);
    x_min = min(x_values);
    y_max = max(y_values);

    %% 실좌표 → 인덱스 변환
    toGrid = @(x, y) [(x - x_min)/resolution + 1, (y_max - y)/resolution + 1];

    start_grid = toGrid(startPose(1), startPose(2));
    goal_grid  = toGrid(goalPose(1), goalPose(2));

    %% 트리 초기화 (모든 노드는 인덱스 좌표로 유지)
    nodes = struct('x', start_grid(1), 'y', start_grid(2), ...
                   'parent', 0, 'cost', 0);

    %% 경로 및 출력 초기화
    path   = struct('x', {}, 'y', {}, 'parent', {}, 'cost', {});
    x_path = zeros(maxPathLength, 1);
    y_path = zeros(maxPathLength, 1);

    %% RRT* 메인 루프 (모든 연산 인덱스 기반)
    for iter = 1:maxIter
        if rand < goalSampleRate
            xr = goal_grid;
        else
            xr = [randi([1, size(map,2)]), randi([1, size(map,1)])];
        end

        [nearestIdx, nearXY] = findNearest(nodes, xr);
        theta = atan2(xr(2)-nearXY(2), xr(1)-nearXY(1));
        newXY = nearXY + stepSize * [cos(theta), sin(theta)];

        if isCollision(newXY, map) || ...
           isPathCollision(nearXY, newXY, map, collisionRes) || ...
           isNearObstacle(newXY, map, safetyDist)
            continue;
        end

        nearIdxs = findNearNodes(nodes, newXY, searchRadius);
        minCost   = nodes(nearestIdx).cost + norm(newXY - nearXY);
        minParent = nearestIdx;

        for idx = 1:numel(nearIdxs)
            iNode = nearIdxs(idx);
            pxy   = [nodes(iNode).x, nodes(iNode).y];
            if ~isPathCollision(pxy, newXY, map, collisionRes)
                c = nodes(iNode).cost + norm(newXY - pxy);
                if c < minCost
                    minCost   = c;
                    minParent = iNode;
                end
            end
        end

        newNode = struct('x', newXY(1), 'y', newXY(2), ...
                         'parent', minParent, 'cost', minCost);
        nodes(end+1) = newNode;
        newIdx       = numel(nodes);

        for idx = 1:numel(nearIdxs)
            iNode = nearIdxs(idx);
            pxy   = [nodes(iNode).x, nodes(iNode).y];
            c     = newNode.cost + norm([newNode.x, newNode.y] - pxy);
            if c < nodes(iNode).cost && ...
               ~isPathCollision([newNode.x,newNode.y], pxy, map, collisionRes)
                nodes(iNode).parent = newIdx;
                nodes(iNode).cost   = c;
            end
        end

        if visualize
            plot([nodes(newNode.parent).x, newNode.x], ...
                 [nodes(newNode.parent).y, newNode.y], '-r');
            hold on;
        end

        if norm(newXY - goal_grid) < successDistTh
            if visualize, disp('[-] GOAL REACHED'); end
            path = backtrace(nodes, newIdx);
            break;
        end
    end

    %% 결과 경로 반환 (인덱스 → 실좌표로 역변환)
    nPath = min(numel(path), maxPathLength);
    x_path_cached = zeros(maxPathLength, 1);
    y_path_cached = zeros(maxPathLength, 1);
    for k = 1:nPath
        x_path_cached(k) = (path(k).x - 1) * resolution + x_min;
        y_path_cached(k) = y_max - (path(k).y - 1) * resolution;
    end

    nPath_cached = nPath;
    path_initialized = true;

    %% === Lightweight Smoothing for Simulink Compatibility ===
    smooth_window = 15;  % 홀수 추천
    if nPath >= smooth_window
        x = x_path_cached(1:nPath);
        y = y_path_cached(1:nPath);

        x_smooth = movmean(x, smooth_window);
        y_smooth = movmean(y, smooth_window);

        % 재샘플링 (고정된 개수로)
        smoothN = 100;
        idx_original = linspace(1, numel(x_smooth), smoothN);
        x_path = interp1(1:numel(x_smooth), x_smooth, idx_original, 'linear')';
        y_path = interp1(1:numel(y_smooth), y_smooth, idx_original, 'linear')';
    else
        x_path = x_path_cached(1:nPath);
        y_path = y_path_cached(1:nPath);
    end


end

%% ======= 서브 함수들 =======

function [idx, xy] = findNearest(nodes, sampleXY)
    d = arrayfun(@(n) hypot(n.x - sampleXY(1), n.y - sampleXY(2)), nodes);
    [~, idx] = min(d);
    xy = [nodes(idx).x, nodes(idx).y];
end

function nearIdxs = findNearNodes(nodes, pos, radius)
    maxNodes = 1000;
    nearIdxs = zeros(1, maxNodes);
    count = 0;
    for i = 1:numel(nodes)
        if hypot(nodes(i).x - pos(1), nodes(i).y - pos(2)) <= radius
            count = count + 1;
            nearIdxs(count) = i;
        end
    end
    nearIdxs = nearIdxs(1:count);
end

function flag = isCollision(pt, map)
    x = round(pt(1)); y = round(pt(2));
    flag = x < 1 || x > size(map,2) || y < 1 || y > size(map,1) || map(y,x) == 1;
end

function flag = isPathCollision(p1, p2, map, step)
    dist = norm(p2 - p1);
    N = max(1, ceil(dist / step));
    flag = false;
    for i = 0:N
        pt = p1 + (p2 - p1) * (i / N);
        if isCollision(pt, map)
            flag = true; return;
        end
    end
end

function flag = isNearObstacle(pt, map, safeDist)
    x0 = round(pt(1)); y0 = round(pt(2));
    r  = ceil(safeDist);
    [X, Y] = meshgrid((x0 - r):(x0 + r), (y0 - r):(y0 + r));
    D2 = (X - pt(1)).^2 + (Y - pt(2)).^2;
    mask = D2 <= safeDist^2;
    X = X(mask); Y = Y(mask);
    valid = X >= 1 & X <= size(map,2) & Y >= 1 & Y <= size(map,1);
    flag  = any(map(sub2ind(size(map), Y(valid), X(valid))) == 1);
end

function path = backtrace(nodes, idx)
    maxPathLen = 500;
    dummyNode = struct('x', 0, 'y', 0, 'parent', 0, 'cost', 0);
    path = repmat(dummyNode, maxPathLen, 1);
    count = 0;
    while idx ~= 0 && count < maxPathLen
        count = count + 1;
        path(count) = nodes(idx);
        idx = nodes(idx).parent;
    end
    path = path(count:-1:1);
end

== stateflow chart generic_IVS/CarMaker/Subsystem/Day3/Chart ==
  (default) -> (junction 1)
  (junction 1) -> (junction 3) [order 1] : [i<99]
      | {i = i + 1;}
  (junction 1) -> (junction 7) [order 2] : {i=0;}
  (junction 3) -> (junction 5)
  (junction 5) -> (junction 7)
  (junction 7) -> (junction 10)
  (junction 10) -> (junction 12) [order 1] : [rem(i,50) == 0]
      | {do_Logic;}
  (junction 10) -> (junction 18) [order 2]
  (junction 12) -> (junction 16)
  (junction 16) -> (junction 18)
  (junction 18) -> (junction 21)
  data: i local =0
  events: do_Logic output FUNCTION_CALL_EVENT

== matlab function generic_IVS/CarMaker/Subsystem/Final Project/Scenario 1/MATLAB Function1 ==
  settings: sampleTime=0.1
  data: u1 input; y output; u2 input
function y = longitudinal_speed_pd_controller_(u1, u2)
    y = 0;
end

== matlab function generic_IVS/CarMaker/Subsystem/Final Project/Scenario 1/MATLAB Function2 ==
  settings: sampleTime=0.1
  data: u input; y output
function y = lateral_pid_controller_(u)
    y = 0;
end
